simulink model "UART"  (R2025a)
settings: Solver=FixedStepAuto  StartTime=0.0  StopTime=10  FixedStep=1e-6  RelTol=1e-3
undefined symbols (not defined in the file): Bit_1, Bit_2, Bit_3, Bit_4, Bit_5, Bit_6, Bit_7, Bit_8
libraries: simulink_extras x158, fl_lib x17, nesl_utility x8, simulink x7
(part 1 of 6)
settings Model: PacingRate=0.010000  Creator=Erys  LastModifiedBy=Erys
settings SolverCC: AllowMultiTaskInputOutput=on

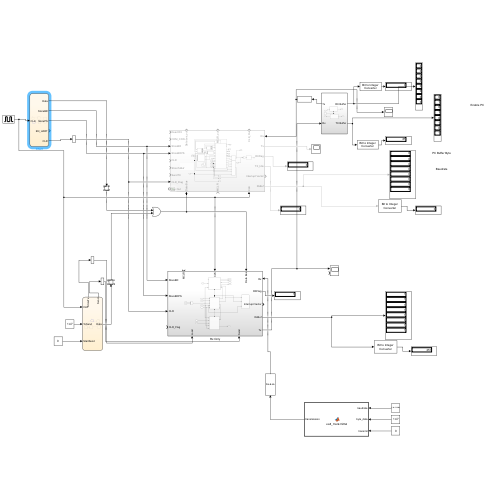
[thumbnail: Simulink's stored preview of the top-level diagram]
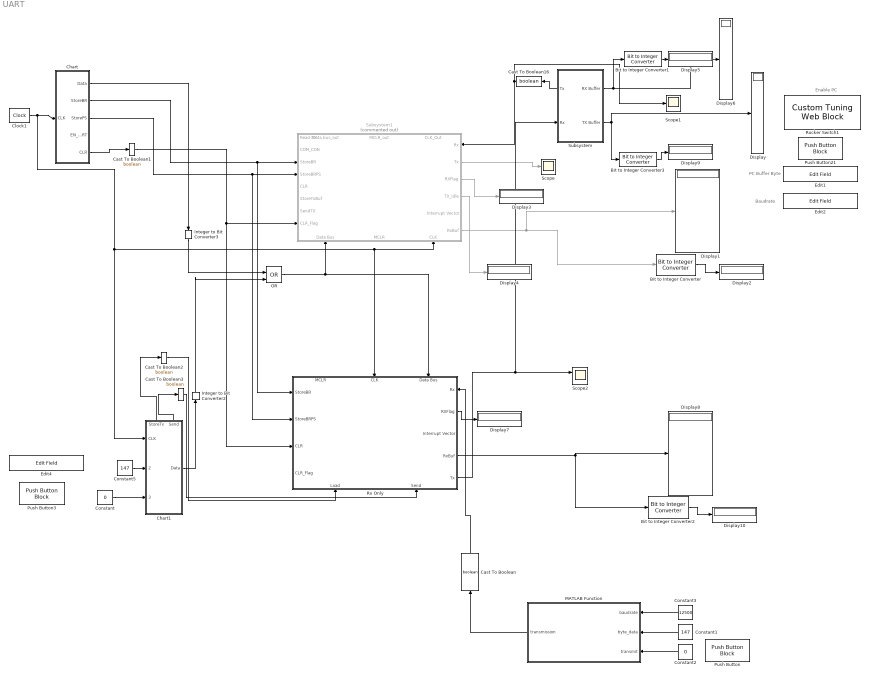
== system UART ==
  note: Enable PC
  note: Baudrate
  note: PC Buffer Byte
  Bit to Integer Converter{,1..3} (4 alike) : simulink/Logic and Bit Operations/Bit to Integer Converter  nbits=8  bitOrder=MSB first  signedOutputValues=Unsigned  outDtype=Inherit via internal rule  outDtypeSigned=Inherit via internal rule
  Cast To Boolean{,1..3,16} (5 alike) : DataTypeConversion  OutDataTypeStr=boolean  SaturateOnIntegerOverflow=off  RndMeth=Floor
  Chart : Stateflow chart  TreatAsAtomicUnit=on
      settings: PortSchema="{\"entries\":[{\"content\":{\"sides\":[{\"content\":{\"connectorIds\":[\"In1\"]},\"type\":\"ConnectorPlacement.EquallySpacedRectSide\",\"uuid\":\"579546ec-ba1d-42e0-bb7d-99479c6f4574\"},{\"content\":{\"connectorIds\":[\"Out2\",\"Out3\",\"Out4\",\"Out5\",\"Out1\"],\"side\":\"RIGHT\"},\"type\":\"ConnectorPlacement.EquallySpacedRectSide\",\"uuid\":\"86ca8068-8b90-4ed4-9903-80afb514b4dd\"},{\"content\":{\"side\":\"TOP\"},\"type\":\"ConnectorPlacement.EquallySpacedRectSide\",\"uuid\":\"acfe83ec-086c-472c-903c-42e246259d52\"}]},\"type\":\"ConnectorPlacement.EquallySpacedConnector\",\"uuid\":\"539fa3bb-c07f-4066-9107-75efb32f7eda\"}],\"packageUris\":[\"http://schema.mathworks.com/mf0/Connector/R2020b\"],\"version\":\"1.0\"}"
  Chart1 : Stateflow chart  TreatAsAtomicUnit=on
      settings: PortSchema="{\"entries\":[{\"content\":{\"sides\":[{\"content\":{\"connectorIds\":[\"In1\",\"In2\",\"In3\"]},\"type\":\"ConnectorPlacement.EquallySpacedRectSide\",\"uuid\":\"579546ec-ba1d-42e0-bb7d-99479c6f4574\"},{\"content\":{\"connectorIds\":[\"Out1\"],\"side\":\"RIGHT\"},\"type\":\"ConnectorPlacement.EquallySpacedRectSide\",\"uuid\":\"86ca8068-8b90-4ed4-9903-80afb514b4dd\"},{\"content\":{\"connectorIds\":[\"Out2\",\"Out3\"],\"side\":\"TOP\"},\"type\":\"ConnectorPlacement.EquallySpacedRectSide\",\"uuid\":\"acfe83ec-086c-472c-903c-42e246259d52\"}]},\"type\":\"ConnectorPlacement.EquallySpacedConnector\",\"uuid\":\"539fa3bb-c07f-4066-9107-75efb32f7eda\"}],\"packageUris\":[\"http://schema.mathworks.com/mf0/Connector/R2020b\"],\"version\":\"1.0\"}"
  Clock1 : simulink_extras/Flip Flops/Clock  period=0.00001
  Constant : Constant  Value=0
  Constant1 : Constant  Value=147
  Constant2 : Constant  Value=0
  Constant3 : Constant  Value=12500
  Constant5 : Constant  Value=147  OutDataTypeStr=double
  Display{,1..10} (11 alike) : Display
  Edit1 : EditField  LabelPosition=Hide  ShowInitialText=on  Alignment=Center
  Edit2 : EditField  LabelPosition=Hide  ShowInitialText=on  Alignment=Center
  Edit4 : EditField  LabelPosition=Hide  ShowInitialText=on  Alignment=Center
  Integer to Bit Converter2 : simulink/Logic and Bit Operations/Integer to Bit Converter  nbits=8  signedInputValues=Unsigned  bitOrder=MSB first  outDtype=Inherit via internal rule
  Integer to Bit Converter3 : simulink/Logic and Bit Operations/Integer to Bit Converter  nbits=8  signedInputValues=Unsigned  bitOrder=MSB first  outDtype=Inherit via internal rule
  MATLAB Function : MATLAB Function  TreatAsAtomicUnit=on
  OR : Logic  Operator=OR  IconShape=distinctive  AllPortsSameDT=off  OutDataTypeStr=boolean
  Push Button : PushButtonBlock  IconOnColor=[0.0, 0.39215686274509803, 0.0]  IconOffColor=[0.0, 1.0, 0.0]  OffValue=0.000000
  Push Button21 : PushButtonBlock  ButtonText=Send  IconOnColor=[0.0, 0.39215686274509803, 0.0]  IconOffColor=[0.0, 1.0, 0.0]  OffValue=0.000000
  Push Button3 : PushButtonBlock  ButtonText=Send  ButtonType=Latch  IconOnColor=[0.0, 0.39215686274509803, 0.0]  IconOffColor=[0.0, 1.0, 0.0]  OffValue=0.000000
  Rocker Switch1 : CustomTuningWebBlock  LabelPosition=Hide  ShowInitialText=on  Configuration="{\"components\":[{\"name\":\"CustomSwitchStateComponent\",\"settings\":{\"position\":[0,0,1,1],\"states\":[{\"HitRegion\":{\"position\":[0,0,0.5,1]},\"Image\":{\"position\":[0.13,0,1,0.75],\"size\":[1,0.75],\"src\":\"data:image\\/svg+xml;base64,PHN2ZyB4bWxucz0iaHR0cDovL3d3dy53My5vcmcvMjAwMC9zdmciIHhtbG5zOnhsaW5rPSJodHRwOi8vd3d3LnczLm9yZy8xOTk5L3hsaW5rIiB2aWV3Qm94PSIwIDAgNzUgMjQuOCI+PGRlZnM+PHN0eWxlPi5jbHMtMXtmaWxsOnVybCgjcmFkaWFsLWdyYWRpZW50KTt9LmNscy0ye2ZpbGw6dXJsKCNyYWRpYWwtZ3JhZGllbnQtMik7fS5jbHMtM3tzdHJva2U6I2IyMDAwMDtzdHJva2Utd2lkdGg6MC4yNXB4O2ZpbGw6dXJsKCNsaW5lYXItZ3JhZGllbnQpO30uY2xzLTR7ZmlsbDp1cmwoI2xpbmVhci1ncmFkaWVudC0yKTt9LmNs ...(+3576 chars)\",\"srcOrientation\":\"Right\"},\"Label\":{\"color\":[0.5019607843137255,0.5019607843137255,0.5019607843137255],\"icon\":{\"size\":[0,0],\"src\":[],\"srcOrientation\":\"Right\"},\"iconPlacement\":\"left\",\"opacity\":1,\"position\":[0.5,0.08],\"show\":true,\"text\":{\"content\":\"Off\",\"font\":\"Helvetica\"}},\"Value\":0},{\"HitRegion\":{\"position\":[0,0.5,0.5,1]},\"Image\":{\"position\":[0.13,0,1,0.75],\"size\":[1,0.75],\"src\":\"data:image\\/svg+xml;base64,PHN2ZyB4bWxucz0iaHR0cDovL3d3dy53My5vcmcvMjAwMC9zdmciIHhtbG5zOnhsaW5rPSJodHRwOi8vd3d3LnczLm9yZy8xOTk5L3hsaW5rIiB2aWV3Qm94PSIwIDAgNzUgMjQuOCI+PGRlZnM+PHN0eWxlPi5jbHMtMXtmaWxsOnVybCgjcmFkaWFsLWdyYWRpZW50KTt9LmNscy0ye2ZpbGw6dXJsKCNyYWRpYWwtZ3JhZGllbnQtMik7fS5jbHMtM3tzdHJva2U6I2IyMDAwMDtzdHJva2Utd2lkdGg6MC4yNXB4O2ZpbGw6dXJsKCNsaW5lYXItZ3JhZGllbnQpO30uY2xzLTR7ZmlsbDp1cmwoI2xpbmVhci1ncmFkaWVudC0yKTt9LmNs ...(+3520 chars)\",\"srcOrientation\":\"Right\"},\"Label\":{\"color\":[0.5019607843137255,0.5019607843137255,0.5019607843137255],\"icon\":{\"size\":[0,0],\"src\":[],\"srcOrientation\":\"Right\"},\"iconPlacement\":\"left\",\"opacity\":1,\"position\":[0.5,0.92],\"show\":true,\"text\":{\"content\":\"On\",\"font\":\"Helvetica\"}},\"Value\":1}]}},{\"name\":\"BackgroundImageComponent\",\"settings\":{\"image\":{\"size\":[155,70],\"src\":\"default\",\"srcOrientation\":\"Right\"},\"position\":[0,0,1,1],\"scaleMode\":\"0\"}},{\"name\":\"ForegroundImageComponent\",\"settings\":{\"image\":{\"size\":[0,0],\"src\":\"default\",\"srcOrientation\":[]},\"isForeground\":1,\"position\":[0,0,1,1],\"scaleMode\":\"0\"}}],\"derived\":{\"blockParameters\":{\"StatesJSON\":[{\"Label\":\"Off\",\"Value\":0},{\"Label\":\"On\",\"Value\":1}],\"fixedAspectRatio\":\"on\"}},\"settings\":{\"BindingType\":\"param\",\"backgroundColor\":[0,0,255,\"1\"],\"backgroundOffset\":0.14,\"fixedAspectRatio\":\"on\",\"foregroundColor\":[234,234,234],\"showBackgroundColor\":false,\"variant\":\"rocker\",\"version\":\"R2024b\"},\"type\":\"Switch\"}"
  Rx Only : Subsystem
      settings: PortSchema="{\"entries\":[{\"content\":{\"sides\":[{\"content\":{\"connectorIds\":[\"In1\",\"In2\",\"In3\",\"In4\"]},\"type\":\"ConnectorPlacement.EquallySpacedRectSide\",\"uuid\":\"e85603b6-4ed5-4461-b09c-fd6c21df1c06\"},{\"content\":{\"connectorIds\":[\"In10\",\"Out1\",\"Out2\",\"Out3\",\"Out4\"],\"side\":\"RIGHT\"},\"type\":\"ConnectorPlacement.EquallySpacedRectSide\",\"uuid\":\"5db2c6ff-63a0-4798-8f8b-4dedc9cdcacf\"},{\"content\":{\"connectorIds\":[\"In5\",\"In6\",\"In7\"],\"side\":\"TOP\"},\"type\":\"ConnectorPlacement.EquallySpacedRectSide\",\"uuid\":\"f0c8188e-88ef-4c96-9e6b-84318d61a16d\"},{\"content\":{\"connectorIds\":[\"In8\",\"In9\"],\"side\":\"BOTTOM\"},\"type\":\"ConnectorPlacement.EquallySpacedRectSide\",\"uuid\":\"72c99dac-0a0c-46d1-ab81-9f63741ecdc0\"}]},\"type\":\"ConnectorPlacement.EquallySpacedConnector\",\"uuid\":\"b744ad23-58d2-4187-a0b7-9a75f0b078d3\"}],\"packageUris\":[\"http://schema.mathworks.com/mf0/Connector/R2020b\"],\"version\":\"1.0\"}"
  Scope : Scope
      settings: ActiveDisplayYMinimum=-1  ActiveDisplayYMaximum=1
  Scope1 : Scope
      settings: ActiveDisplayYMinimum=-0.125  ActiveDisplayYMaximum=1.125
  Scope2 : Scope  NumInputPorts=2
      settings: ActiveDisplayYMinimum=0.9  ActiveDisplayYMaximum=1.1
  Subsystem : Subsystem
      settings: PortSchema="{\"entries\":[{\"content\":{\"sides\":[{\"content\":{\"connectorIds\":[\"Out3\",\"In1\"]},\"type\":\"ConnectorPlacement.EquallySpacedRectSide\",\"uuid\":\"895b9a17-19e6-4759-8585-1efebccf03ce\"},{\"content\":{\"connectorIds\":[\"Out1\",\"Out2\"],\"side\":\"RIGHT\"},\"type\":\"ConnectorPlacement.EquallySpacedRectSide\",\"uuid\":\"c1f476a2-53d3-43a2-8378-f6bf9a8ea71f\"},{\"content\":{\"side\":\"TOP\"},\"type\":\"ConnectorPlacement.EquallySpacedRectSide\",\"uuid\":\"a179f0e6-f4b5-47af-a583-92dca50b06ef\"}]},\"type\":\"ConnectorPlacement.EquallySpacedConnector\",\"uuid\":\"ea5a564d-b62d-4fb1-ae9a-ba3c651dd29f\"}],\"packageUris\":[\"http://schema.mathworks.com/mf0/Connector/R2020b\"],\"version\":\"1.0\"}"
  Subsystem1 : Subsystem  Commented=on
      settings: PortSchema="{\"entries\":[{\"content\":{\"sides\":[{\"content\":{\"connectorIds\":[\"In1\",\"In2\",\"In3\",\"In4\",\"In5\",\"In6\",\"In7\",\"In8\",\"LConn1\"]},\"type\":\"ConnectorPlacement.EquallySpacedRectSide\",\"uuid\":\"e85603b6-4ed5-4461-b09c-fd6c21df1c06\"},{\"content\":{\"connectorIds\":[\"In12\",\"Out1\",\"Out2\",\"Out3\",\"Out4\",\"Out5\"],\"side\":\"RIGHT\"},\"type\":\"ConnectorPlacement.EquallySpacedRectSide\",\"uuid\":\"5db2c6ff-63a0-4798-8f8b-4dedc9cdcacf\"},{\"content\":{\"connectorIds\":[\"Out6\",\"Out7\",\"Out8\"],\"side\":\"TOP\"},\"type\":\"ConnectorPlacement.EquallySpacedRectSide\",\"uuid\":\"f0c8188e-88ef-4c96-9e6b-84318d61a16d\"},{\"content\":{\"connectorIds\":[\"In9\",\"In10\",\"In11\"],\"side\":\"BOTTOM\"},\"type\":\"ConnectorPlacement.EquallySpacedRectSide\",\"uuid\":\"72c99dac-0a0c-46d1-ab81-9f63741ecdc0\"}]},\"type\":\"ConnectorPlacement.EquallySpacedConnector\",\"uuid\":\"b744ad23-58d2-4187-a0b7-9a75f0b078d3\"}],\"packageUris\":[\"http://schema.mathworks.com/mf0/Connector/R2020b\"],\"version\":\"1.0\"}"
  wires:
  Bit to Integer Converter1/1 -> Display5/1
  Subsystem/1(RX Buffer) -> Display6/1, Bit to Integer Converter1/1
  Subsystem/3(Tx) -> Cast To Boolean16/1
  Subsystem/2(TX Buffer) -> Display/1, Bit to Integer Converter3/1
  Bit to Integer Converter3/1 -> Display9/1
  Clock1/1 -> Subsystem1/11(CLK), Rx Only/6(CLK), Chart1/1(CLK), Chart/1(CLK)
  Bit to Integer Converter/1 -> Display2/1
  Subsystem1/5(RxBuf) -> Display1/1, Bit to Integer Converter/1
  Cast To Boolean16/1 -> Subsystem1/12(Rx), Scope1/1
  Chart/3(StoreBR) -> Rx Only/1(StoreBR), Subsystem1/3(StoreBR)
  Chart/4(StorePS) -> Rx Only/2(StoreBRPS), Subsystem1/4(StoreBRPS)
  Chart/1(CLR) -> Cast To Boolean1/1
  Chart1/3(Send) -> Cast To Boolean3/1
  Cast To Boolean1/1 -> Rx Only/3(CLR), Subsystem1/8(CLR_Flag)
  Subsystem1/1(Tx) -> Scope/1
  Chart1/1(Data) -> Integer to Bit Converter2/1
  Chart1/2(StoreTx) -> Cast To Boolean2/1
  Constant5/1 -> Chart1/2(ToSend)
  Constant/1 -> Chart1/3(StartSend)
  Integer to Bit Converter2/1 -> OR/2
  Chart/2(Data) -> Integer to Bit Converter3/1
  OR/1 -> Rx Only/7(Data Bus), Subsystem1/9(Data Bus)
  Integer to Bit Converter3/1 -> OR/1
  Subsystem1/2(RXFlag) -> Display3/1
  Subsystem1/3(TX_Idle) -> Display4/1
  Rx Only/1(RXFlag) -> Display7/1
  Bit to Integer Converter2/1 -> Display10/1
  Rx Only/3(RxBuf) -> Display8/1, Bit to Integer Converter2/1
  Constant1/1 -> MATLAB Function/2(byte_data)
  Constant3/1 -> MATLAB Function/1(baudrate)
  Constant2/1 -> MATLAB Function/3(transmit)
  MATLAB Function/1(transmission) -> Cast To Boolean/1
  Cast To Boolean3/1 -> Rx Only/9(Send)
  Cast To Boolean2/1 -> Rx Only/8(Load)
  Rx Only/4(Tx) -> Scope2/1, Subsystem/1(Rx)
  Cast To Boolean/1 -> Rx Only/10(Rx)

== system UART/Rx Only ==
  StoreBR : Inport
  StoreBRPS : Inport  Port=2
  CLR : Inport  Port=3
  CLR_Flag : Inport  Port=4
  MCLR : Inport  Port=5
  CLK : Inport  Port=6
  Data Bus : Inport  Port=7
  Load : Inport  Port=8
  Send : Inport  Port=9
  Rx : Inport  Port=10
  Baudrate Generator : Subsystem
      settings: PortSchema="{\"entries\":[{\"content\":{\"sides\":[{\"content\":{\"connectorIds\":[\"In1\",\"In2\",\"In3\",\"In4\",\"In5\"]},\"type\":\"ConnectorPlacement.EquallySpacedRectSide\",\"uuid\":\"d194f446-ff7e-400e-97b6-75d09d731b88\"},{\"content\":{\"connectorIds\":[\"Out1\",\"Out2\",\"Out3\",\"Out4\"],\"side\":\"RIGHT\"},\"type\":\"ConnectorPlacement.EquallySpacedRectSide\",\"uuid\":\"c109133b-911d-4f42-82c9-f4bf3d965687\"},{\"content\":{\"connectorIds\":[\"In6\"],\"side\":\"TOP\"},\"type\":\"ConnectorPlacement.EquallySpacedRectSide\",\"uuid\":\"a9d3f627-7d58-48c5-bb3c-ddb572323ed2\"},{\"content\":{\"connectorIds\":[\"In7\"],\"side\":\"BOTTOM\"},\"type\":\"ConnectorPlacement.EquallySpacedRectSide\",\"uuid\":\"95ca91ff-0310-4968-b6f0-040fa48d6210\"}]},\"type\":\"ConnectorPlacement.EquallySpacedConnector\",\"uuid\":\"72d75e6a-49d5-4268-b431-51d3f4095294\"}],\"packageUris\":[\"http://schema.mathworks.com/mf0/Connector/R2020b\"],\"version\":\"1.0\"}"
  OR4 : Logic  Operator=OR  IconShape=distinctive  AllPortsSameDT=off  OutDataTypeStr=boolean
  Scope : Scope  NumInputPorts=3
      settings: ActiveDisplayString=3  ActiveDisplayYMinimum=-0.12499999999999997  ActiveDisplayYMaximum=1.125  DataLoggingVariableName=ScopeData3
  Subsystem1 : Subsystem
      settings: PortSchema="{\"entries\":[{\"content\":{\"sides\":[{\"content\":{\"connectorIds\":[\"In1\",\"In2\",\"In3\"]},\"type\":\"ConnectorPlacement.EquallySpacedRectSide\",\"uuid\":\"26de21f2-c2ce-4306-8005-25e34fc94ef8\"},{\"content\":{\"connectorIds\":[\"Out1\",\"Out2\",\"In4\",\"Out3\",\"In5\",\"In6\"],\"side\":\"RIGHT\"},\"type\":\"ConnectorPlacement.EquallySpacedRectSide\",\"uuid\":\"87f33876-7706-47c8-9618-d671270088cd\"},{\"content\":{\"side\":\"TOP\"},\"type\":\"ConnectorPlacement.EquallySpacedRectSide\",\"uuid\":\"145d03ab-c1b9-4d18-a52c-c9347f9686a8\"},{\"content\":{\"connectorIds\":[\"Out4\"],\"side\":\"BOTTOM\"},\"type\":\"ConnectorPlacement.EquallySpacedRectSide\",\"uuid\":\"eb75dd28-797f-4c73-8962-4db24c637120\"}]},\"type\":\"ConnectorPlacement.EquallySpacedConnector\",\"uuid\":\"6afd2c35-7a81-4ee8-ac82-dba626904bf2\"}],\"packageUris\":[\"http://schema.mathworks.com/mf0/Connector/R2020b\"],\"version\":\"1.0\"}"
  Subsystem2 : Subsystem
      settings: PortSchema="{\"entries\":[{\"content\":{\"sides\":[{\"content\":{\"connectorIds\":[\"In1\",\"In2\",\"In3\",\"In4\",\"In5\"]},\"type\":\"ConnectorPlacement.EquallySpacedRectSide\",\"uuid\":\"1da95ee2-7c6b-483d-95ed-13ac8495d1ed\"},{\"content\":{\"connectorIds\":[\"In6\",\"Out1\"],\"side\":\"RIGHT\"},\"type\":\"ConnectorPlacement.EquallySpacedRectSide\",\"uuid\":\"39299cfc-3cbd-4586-b435-63be24abc51d\"},{\"content\":{\"connectorIds\":[\"Out2\"],\"side\":\"TOP\"},\"type\":\"ConnectorPlacement.EquallySpacedRectSide\",\"uuid\":\"75fe8f74-28fb-448a-b371-b155707b28cf\"}]},\"type\":\"ConnectorPlacement.EquallySpacedConnector\",\"uuid\":\"bfefa0d3-97e8-496e-8e8b-94574003bbd4\"}],\"packageUris\":[\"http://schema.mathworks.com/mf0/Connector/R2020b\"],\"version\":\"1.0\"}"
  RXFlag : Outport
  Interrupt Vector : Outport  Port=2
  RxBuf : Outport  Port=3
  Tx : Outport  Port=4
  wires:
  MCLR/1 -> OR4/2
  OR4/1 -> Subsystem2/1(UARTCLR), Baudrate Generator/3(CLR), Subsystem1/3(UART_CLR)
  CLK/1 -> Scope/3, Baudrate Generator/4(CLK), Subsystem2/4(CLK)
  StoreBRPS/1 -> Baudrate Generator/2(StoreTPS)
  StoreBR/1 -> Baudrate Generator/1(StoreBR)
  Baudrate Generator/2(B_CLK_RX) -> Subsystem1/5(B_CLK), Scope/1  "BAUD CLK"
  CLR/1 -> OR4/1
  Data Bus/1 -> Baudrate Generator/5(Data Bus), Subsystem2/5(Data Bus)
  Send/1 -> Subsystem2/2(SendTX)
  Load/1 -> Subsystem2/3(Load)
  Subsystem2/1(Tx) -> Tx/1
  Baudrate Generator/3(!B_CLK_Tx) -> Subsystem2/6(!B_CLK)
  Rx/1 -> Subsystem1/4(Rx)
  Baudrate Generator/1(!B_CLK_RX) -> Subsystem1/6(!B_CLK)
  CLR_Flag/1 -> Subsystem1/2(CLR_Flag)
  Subsystem1/1(Interrupt Vector) -> Interrupt Vector/1
  Subsystem1/2(Flag) -> RXFlag/1
  Subsystem1/3(RxBuf) -> RxBuf/1
  Subsystem2/2(En_BR) -> Baudrate Generator/7(EnableTx)
  Subsystem1/4(EN_BR) -> Scope/2, Baudrate Generator/6(EnableRx)

== system UART/Subsystem ==
  Rx : Inport
  Constant23 : Constant  Value=12500
  PC RX : Subsystem
      settings: PortSchema="{\"entries\":[{\"content\":{\"sides\":[{\"content\":{\"connectorIds\":[\"In1\"]},\"type\":\"ConnectorPlacement.EquallySpacedRectSide\",\"uuid\":\"5c36fdb9-58e4-4bac-90ea-ae3fb9547746\"},{\"content\":{\"connectorIds\":[\"Out1\"],\"side\":\"RIGHT\"},\"type\":\"ConnectorPlacement.EquallySpacedRectSide\",\"uuid\":\"305a7217-1c2b-4e42-91b3-038d16c5c055\"},{\"content\":{\"side\":\"TOP\"},\"type\":\"ConnectorPlacement.EquallySpacedRectSide\",\"uuid\":\"8bca033e-7423-4813-979e-646ac4ffc9f5\"},{\"content\":{\"connectorIds\":[\"In2\"],\"side\":\"BOTTOM\"},\"type\":\"ConnectorPlacement.EquallySpacedRectSide\",\"uuid\":\"0fb3eda9-6a9e-42f2-8b90-ae90f87eee38\"}]},\"type\":\"ConnectorPlacement.EquallySpacedConnector\",\"uuid\":\"4522f435-3b11-47d6-b8b1-c58661572e67\"}],\"packageUris\":[\"http://schema.mathworks.com/mf0/Connector/R2020b\"],\"version\":\"1.0\"}"
  PC Tx : Subsystem
      settings: PortSchema="{\"entries\":[{\"content\":{\"sides\":[{\"content\":{\"connectorIds\":[\"Out2\"]},\"type\":\"ConnectorPlacement.EquallySpacedRectSide\",\"uuid\":\"4cc81552-4785-4fe1-ba4c-afd427c4a9be\"},{\"content\":{\"connectorIds\":[\"Out1\"],\"side\":\"RIGHT\"},\"type\":\"ConnectorPlacement.EquallySpacedRectSide\",\"uuid\":\"17a0d90d-16da-439e-9c28-79f860db0d72\"},{\"content\":{\"connectorIds\":[\"In1\"],\"side\":\"TOP\"},\"type\":\"ConnectorPlacement.EquallySpacedRectSide\",\"uuid\":\"85a74a21-901d-48e2-982c-d40d9a6c8828\"}]},\"type\":\"ConnectorPlacement.EquallySpacedConnector\",\"uuid\":\"f7431681-2562-4b57-bc58-81cf5712b5b5\"}],\"packageUris\":[\"http://schema.mathworks.com/mf0/Connector/R2020b\"],\"version\":\"1.0\"}"
  RX Buffer : Outport
  TX Buffer : Outport  Port=2
  Tx : Outport  Port=3
  wires:
  Rx/1 -> PC RX/1(Rx)
  PC Tx/2(Tx) -> Tx/1
  PC RX/1(Buffer) -> RX Buffer/1
  PC Tx/1(Buffer) -> TX Buffer/1
  Constant23/1 -> PC Tx/1(Baudrate), PC RX/2(Baudrate)

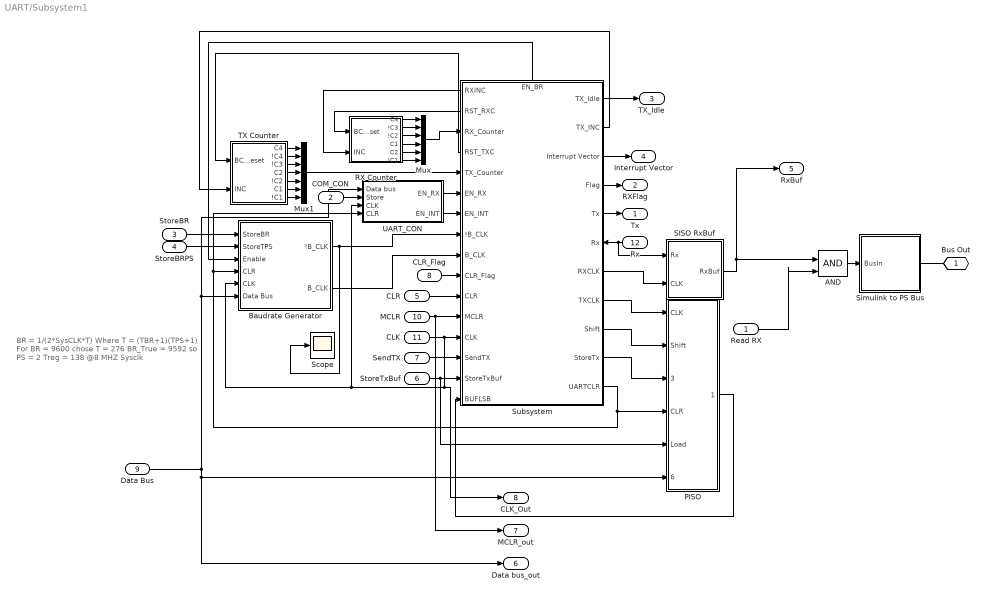
== system UART/Subsystem1 ==
  note: BR = 1/(2*SysCLK*T)
      | Where T = (TBR+1)(TPS+1)
      | For BR = 9600 chose T = 276 BR_True = 9592
      |
      | so PS = 2
      | Treg = 138
      |
      | @8 MHZ Sysclk
  Read RX : Inport
  COM_CON : Inport  Port=2
  StoreBR : Inport  Port=3
  StoreBRPS : Inport  Port=4
  CLR : Inport  Port=5
  StoreTxBuf : Inport  Port=6
  SendTX : Inport  Port=7
  CLR_Flag : Inport  Port=8
  Data Bus : Inport  Port=9
  MCLR : Inport  Port=10
  CLK : Inport  Port=11
  Rx : Inport  Port=12
  AND : Logic  IconShape=distinctive  AllPortsSameDT=off  OutDataTypeStr=boolean
  Baudrate Generator : Subsystem
  Mux : Mux  Inputs=6
  Mux1 : Mux  Inputs=7
  PISO : Subsystem
  RX Counter : Subsystem
  SISO RxBuf : Subsystem
  Scope : Scope
      settings: ActiveDisplayYMinimum=-0.011295344536901064  ActiveDisplayYMaximum=1.0251315467449829
  Simulink to PS Bus : Subsystem
  Subsystem : Subsystem
      settings: PortSchema="{\"entries\":[{\"content\":{\"sides\":[{\"content\":{\"connectorIds\":[\"Out12\",\"Out13\",\"In1\",\"Out14\",\"In2\",\"In3\",\"In4\",\"In5\",\"In6\",\"In7\",\"In8\",\"In9\",\"In10\",\"In11\",\"In12\",\"In13\"]},\"type\":\"ConnectorPlacement.EquallySpacedRectSide\",\"uuid\":\"5f740d6e-15c2-47b5-8101-a8ac2908b9d5\"},{\"content\":{\"connectorIds\":[\"Out1\",\"Out2\",\"Out3\",\"Out4\",\"Out5\",\"In14\",\"Out6\",\"Out7\",\"Out8\",\"Out9\",\"Out10\"],\"side\":\"RIGHT\"},\"type\":\"ConnectorPlacement.EquallySpacedRectSide\",\"uuid\":\"5d214534-1223-4301-a5a7-3ca5e7f086fd\"},{\"content\":{\"connectorIds\":[\"Out11\"],\"side\":\"TOP\"},\"type\":\"ConnectorPlacement.EquallySpacedRectSide\",\"uuid\":\"1d2213ce-2390-4a69-a57b-c28668a5aa5c\"}]},\"type\":\"ConnectorPlacement.EquallySpacedConnector\",\"uuid\":\"5a906a9e-6d2c-4523-95ab-0413fe814690\"}],\"packageUris\":[\"http://schema.mathworks.com/mf0/Connector/R2020b\"],\"version\":\"1.0\"}"
  TX Counter : Subsystem
  UART_CON : Subsystem
  Bus Out : PMIOPort  Side=Left
  Tx : Outport
  RXFlag : Outport  Port=2
  TX_Idle : Outport  Port=3
  Interrupt Vector : Outport  Port=4
  RxBuf : Outport  Port=5
  Data bus_out : Outport  Port=6
  MCLR_out : Outport  Port=7
  CLK_Out : Outport  Port=8
  wires:
  MCLR/1 -> MCLR_out/1, Subsystem/9(MCLR)
  UART_CON/1(EN_RX) -> Subsystem/3(EN_RX)
  UART_CON/2(EN_INT) -> Subsystem/4(EN_INT)
  COM_CON/1 -> UART_CON/2(Store)
  SendTX/1 -> Subsystem/11(SendTX)
  CLR_Flag/1 -> Subsystem/7(CLR_Flag)
  Data Bus/1 -> PISO/6(Data Bus), Data bus_out/1, Baudrate Generator/6(Data Bus), UART_CON/1(Data bus)
  StoreTxBuf/1 -> Subsystem/12(StoreTxBuf), PISO/5(Load)
  Subsystem/13(RST_RXC) -> RX Counter/1(BC_Reset)
  Subsystem/9(StoreTx) -> PISO/3(Store TXBUF)
  Subsystem/2(TX_INC) -> TX Counter/2(INC)
  Subsystem/14(RST_TXC) -> TX Counter/1(BC_Reset)
  Subsystem/4(Flag) -> RXFlag/1
  Subsystem/3(Interrupt Vector) -> Interrupt Vector/1
  Subsystem/12(RXINC) -> RX Counter/2(INC)
  Subsystem/10(UARTCLR) -> UART_CON/4(CLR), Baudrate Generator/4(CLR), PISO/4("CLR ")
  Rx/1 -> SISO RxBuf/1(Rx), Subsystem/14(Rx)
  CLK/1 -> Subsystem/10(CLK), CLK_Out/1, Baudrate Generator/5(CLK), UART_CON/3(CLK)
  Subsystem/5(Tx) -> Tx/1
  Subsystem/7(TXCLK) -> PISO/1("CLK ")
  Subsystem/11(EN_BR) -> Baudrate Generator/3(Enable)
  Subsystem/8(Shift) -> PISO/2(Shift)
  StoreBRPS/1 -> Baudrate Generator/2(StoreTPS)
  StoreBR/1 -> Baudrate Generator/1(StoreBR)
  SISO RxBuf/1(RxBuf) -> RxBuf/1, AND/1
  PISO/1(Serial_out) -> Subsystem/13(BUFLSB)
  Baudrate Generator/2(B_CLK) -> Subsystem/6(B_CLK)
  Baudrate Generator/1(!B_CLK) -> Scope/1, Subsystem/5(!B_CLK)
  RX Counter/1(C4) -> Mux/1
  RX Counter/2(!C3) -> Mux/2
  RX Counter/3(!C2) -> Mux/3
  RX Counter/4(C1) -> Mux/4
  Mux/1 -> Subsystem/1(RX_Counter)
  TX Counter/1(C4) -> Mux1/1
  TX Counter/2(!C4) -> Mux1/2
  TX Counter/3(!C3) -> Mux1/3
  TX Counter/4(C2) -> Mux1/4
  TX Counter/5(!C2) -> Mux1/5
  TX Counter/6(C1) -> Mux1/6
  TX Counter/7(!C1) -> Mux1/7
  Mux1/1 -> Subsystem/2(TX_Counter)
  CLR/1 -> Subsystem/8(CLR)
  Subsystem/1(TX_Idle) -> TX_Idle/1
  Read RX/1 -> AND/2
  AND/1 -> Simulink to PS Bus/1(BusIn)
  RX Counter/5(C2) -> Mux/5
  RX Counter/6(!C1) -> Mux/6
  Subsystem/6(RXCLK) -> SISO RxBuf/2(CLK)
  connections:
  Bus Out/RConn1 -- Simulink to PS Bus/RConn1

== system UART/Rx Only/Baudrate Generator ==
  StoreBR : Inport
  StoreTPS : Inport  Port=2
  CLR : Inport  Port=3
  CLK : Inport  Port=4
  Data Bus : Inport  Port=5
  EnableRx : Inport  Port=6
  EnableTx : Inport  Port=7
  BPS : Subsystem
  BR : Subsystem
  BaudTimer : Subsystem
  BaudTimer1 : Subsystem
  !B_CLK_RX : Outport
  B_CLK_RX : Outport  Port=2
  !B_CLK_Tx : Outport  Port=3
  B_CLK_Tx : Outport  Port=4
  wires:
  CLK/1 -> BaudTimer/7(CLK), BaudTimer1/7(CLK), BR/3(CLK), BPS/3(CLK)
  StoreBR/1 -> BaudTimer/1(StoreBR), BaudTimer1/1(StoreBR), BR/2(Store)
  Data Bus/1 -> BPS/1(Data bus), BR/1(Data bus)
  CLR/1 -> BaudTimer1/4("CLR "), BPS/4(CLR), BaudTimer/4("CLR "), BR/4(CLR)
  StoreTPS/1 -> BaudTimer/5(StorePS), BaudTimer1/5(StorePS), BPS/2(Store)
  BR/1("Q Bus ") -> BaudTimer/2(BR_Reg), BaudTimer1/2(BR_Reg)
  EnableRx/1 -> BaudTimer/3(Enable)
  BPS/1("Q Bus ") -> BaudTimer/6(TReg), BaudTimer1/6(TReg)
  BaudTimer/2(!B_CLK) -> !B_CLK_RX/1
  BaudTimer/1(B_CLK) -> B_CLK_RX/1
  EnableTx/1 -> BaudTimer1/3(Enable)
  BaudTimer1/2(!B_CLK) -> !B_CLK_Tx/1
  BaudTimer1/1(B_CLK) -> B_CLK_Tx/1

== system UART/Rx Only/Subsystem1 ==
  EN_INT : Inport
  CLR_Flag : Inport  Port=2
  UART_CLR : Inport  Port=3
  Rx : Inport  Port=4
  B_CLK : Inport  Port=5
  !B_CLK : Inport  Port=6
  Constant : Constant
  Mux : Mux
  RX Counter : Subsystem
  SIPO RxBuf : Subsystem
  Subsystem : Subsystem
      settings: PortSchema="{\"entries\":[{\"content\":{\"sides\":[{\"content\":{\"connectorIds\":[\"Out5\",\"Out6\",\"In1\",\"In2\",\"In3\",\"In4\",\"In5\",\"In6\"]},\"type\":\"ConnectorPlacement.EquallySpacedRectSide\",\"uuid\":\"5f740d6e-15c2-47b5-8101-a8ac2908b9d5\"},{\"content\":{\"connectorIds\":[\"Out1\",\"Out2\",\"In8\",\"Out3\"],\"side\":\"RIGHT\"},\"type\":\"ConnectorPlacement.EquallySpacedRectSide\",\"uuid\":\"5d214534-1223-4301-a5a7-3ca5e7f086fd\"},{\"content\":{\"connectorIds\":[\"Out4\"],\"side\":\"TOP\"},\"type\":\"ConnectorPlacement.EquallySpacedRectSide\",\"uuid\":\"1d2213ce-2390-4a69-a57b-c28668a5aa5c\"},{\"content\":{\"connectorIds\":[\"In7\"],\"side\":\"BOTTOM\"},\"type\":\"ConnectorPlacement.EquallySpacedRectSide\",\"uuid\":\"8027d3ec-90e1-4e8c-832f-866f1decbd3b\"}]},\"type\":\"ConnectorPlacement.EquallySpacedConnector\",\"uuid\":\"5a906a9e-6d2c-4523-95ab-0413fe814690\"}],\"packageUris\":[\"http://schema.mathworks.com/mf0/Connector/R2020b\"],\"version\":\"1.0\"}"
  Interrupt Vector : Outport
  Flag : Outport  Port=2
  RxBuf : Outport  Port=3
  EN_BR : Outport  Port=4
  wires:
  Rx/1 -> SIPO RxBuf/1(Rx), Subsystem/8(Rx)
  Constant/1 -> Subsystem/2(EN_RX)
  Subsystem/5(RXINC) -> RX Counter/2(INC)
  EN_INT/1 -> Subsystem/3(EN_INT)
  Subsystem/2(Flag) -> Flag/1
  RX Counter/2(!C3) -> Mux/2
  RX Counter/3(!C2) -> Mux/3
  RX Counter/4(C1) -> Mux/4
  Subsystem/3(RXCLK) -> SIPO RxBuf/2(CLK)
  Subsystem/4(EN_BR) -> EN_BR/1
  RX Counter/1(C4) -> Mux/1
  Subsystem/6(RST_RXC) -> RX Counter/1(BC_Reset)
  Mux/1 -> Subsystem/1(RX_Counter)
  UART_CLR/1 -> Subsystem/7(UART_CLR)
  !B_CLK/1 -> Subsystem/4(!B_CLK)
  Subsystem/1(Interrupt Vector) -> Interrupt Vector/1
  SIPO RxBuf/1(RxBuf) -> RxBuf/1
  CLR_Flag/1 -> Subsystem/6(CLR_Flag)
  B_CLK/1 -> Subsystem/5(B_CLK)

== system UART/Rx Only/Subsystem2 ==
  UARTCLR : Inport
  SendTX : Inport  Port=2
  Load : Inport  Port=3
  CLK : Inport  Port=4
  Data Bus : Inport  Port=5
  !B_CLK : Inport  Port=6
  Mux1 : Mux
  PISO : Subsystem
      settings: PortSchema="{\"entries\":[{\"content\":{\"sides\":[{\"content\":{\"connectorIds\":[\"In1\",\"In2\",\"Out1\",\"In3\",\"In4\"]},\"type\":\"ConnectorPlacement.EquallySpacedRectSide\",\"uuid\":\"1a70dc94-6fd8-45e6-a964-690408e545a5\"},{\"content\":{\"side\":\"RIGHT\"},\"type\":\"ConnectorPlacement.EquallySpacedRectSide\",\"uuid\":\"0446f59e-5565-4f21-b86e-aa6a6c358594\"},{\"content\":{\"connectorIds\":[\"In5\",\"In6\"],\"side\":\"TOP\"},\"type\":\"ConnectorPlacement.EquallySpacedRectSide\",\"uuid\":\"b3251efb-1b02-4ea6-9880-a7aeacd90048\"}]},\"type\":\"ConnectorPlacement.EquallySpacedConnector\",\"uuid\":\"49ea71c8-7b9a-4520-8019-77c12bbc3963\"}],\"packageUris\":[\"http://schema.mathworks.com/mf0/Connector/R2020b\"],\"version\":\"1.0\"}"
  RX Counter1 : Subsystem
  Subsystem1 : Subsystem
      settings: PortSchema="{\"entries\":[{\"content\":{\"sides\":[{\"content\":{\"connectorIds\":[\"Out5\",\"Out6\",\"In1\",\"In2\",\"In3\",\"In4\",\"In5\"]},\"type\":\"ConnectorPlacement.EquallySpacedRectSide\",\"uuid\":\"5f740d6e-15c2-47b5-8101-a8ac2908b9d5\"},{\"content\":{\"connectorIds\":[\"Out1\",\"Out2\",\"Out3\",\"In7\"],\"side\":\"RIGHT\"},\"type\":\"ConnectorPlacement.EquallySpacedRectSide\",\"uuid\":\"5d214534-1223-4301-a5a7-3ca5e7f086fd\"},{\"content\":{\"connectorIds\":[\"In6\",\"Out4\"],\"side\":\"TOP\"},\"type\":\"ConnectorPlacement.EquallySpacedRectSide\",\"uuid\":\"1d2213ce-2390-4a69-a57b-c28668a5aa5c\"}]},\"type\":\"ConnectorPlacement.EquallySpacedConnector\",\"uuid\":\"5a906a9e-6d2c-4523-95ab-0413fe814690\"}],\"packageUris\":[\"http://schema.mathworks.com/mf0/Connector/R2020b\"],\"version\":\"1.0\"}"
  Tx : Outport
  En_BR : Outport  Port=2
  wires:
  Subsystem1/5(TX_INC) -> RX Counter1/2(INC)
  Load/1 -> PISO/3(Load), Subsystem1/5(Load)
  RX Counter1/3(C2) -> Mux1/3
  RX Counter1/4(C1) -> Mux1/4
  RX Counter1/2(!C3) -> Mux1/2
  Subsystem1/2(TXCLK) -> PISO/1("TXCLK ")
  PISO/1(Serial_out) -> Subsystem1/7(BUFLSB)
  UARTCLR/1 -> Subsystem1/6(UARTCLR), PISO/6("CLR ")
  Subsystem1/4(EN_BR) -> En_BR/1, PISO/5(Shift)
  Subsystem1/3(StoreTx) -> PISO/2(Store TXBUF)
  Mux1/1 -> Subsystem1/1(TX_Counter)
  Subsystem1/6(TXC_RST) -> RX Counter1/1(BC_Reset)
  RX Counter1/1(C4) -> Mux1/1
  SendTX/1 -> Subsystem1/4(SendTX)
  !B_CLK/1 -> Subsystem1/3(!B_CLK)
  Data Bus/1 -> PISO/4(Data Bus)
  Subsystem1/1(Tx) -> Tx/1
  CLK/1 -> Subsystem1/2(CLK)

== system UART/Subsystem/PC RX ==
  Rx : Inport
  Baudrate : Inport  Port=2
  Chart : Stateflow chart  TreatAsAtomicUnit=on
      settings: PortSchema="{\"entries\":[{\"content\":{\"sides\":[{\"content\":{\"connectorIds\":[\"In2\",\"In3\"]},\"type\":\"ConnectorPlacement.EquallySpacedRectSide\",\"uuid\":\"b3a5cf11-253b-48e1-b27d-ab3568105f2d\"},{\"content\":{\"connectorIds\":[\"Out1\"],\"side\":\"RIGHT\"},\"type\":\"ConnectorPlacement.EquallySpacedRectSide\",\"uuid\":\"d77e3c4d-b760-45fc-afb9-9b4c779c0c28\"},{\"content\":{\"side\":\"TOP\"},\"type\":\"ConnectorPlacement.EquallySpacedRectSide\",\"uuid\":\"3ac6c7a6-9511-4efe-9c6f-68eb6d23e231\"},{\"content\":{\"connectorIds\":[\"In1\"],\"side\":\"BOTTOM\"},\"type\":\"ConnectorPlacement.EquallySpacedRectSide\",\"uuid\":\"e6165016-b8f7-4206-b89f-4a6ce8b56855\"}]},\"type\":\"ConnectorPlacement.EquallySpacedConnector\",\"uuid\":\"e620c1e0-2324-4d91-a922-d923d05fb9d1\"}],\"packageUris\":[\"http://schema.mathworks.com/mf0/Connector/R2020b\"],\"version\":\"1.0\"}"
  Constant24 : Constant
  MATLAB Function : MATLAB Function  TreatAsAtomicUnit=on
  Buffer : Outport
  wires:
  MATLAB Function/1(y) -> Chart/1(Baudrate)
  Baudrate/1 -> MATLAB Function/1(u)
  Rx/1 -> Chart/3(Rx)
  Constant24/1 -> Chart/2(Enable)
  Chart/1(Buffer) -> Buffer/1

== system UART/Subsystem/PC Tx ==
  Baudrate : Inport
  Chart : Stateflow chart  TreatAsAtomicUnit=on
      settings: PortSchema="{\"entries\":[{\"content\":{\"sides\":[{\"content\":{\"connectorIds\":[\"In2\",\"In3\",\"In1\"]},\"type\":\"ConnectorPlacement.EquallySpacedRectSide\",\"uuid\":\"0fdeee4d-f616-4de4-9957-3fe333ba6b50\"},{\"content\":{\"connectorIds\":[\"Out1\"],\"side\":\"RIGHT\"},\"type\":\"ConnectorPlacement.EquallySpacedRectSide\",\"uuid\":\"b9b055cb-ef8e-482e-98e8-65c3605d7f8f\"},{\"content\":{\"connectorIds\":[\"In4\"],\"side\":\"TOP\"},\"type\":\"ConnectorPlacement.EquallySpacedRectSide\",\"uuid\":\"a4fa0ffa-46c2-4446-908b-2de4127fdb17\"}]},\"type\":\"ConnectorPlacement.EquallySpacedConnector\",\"uuid\":\"eba70a97-dbbd-4797-9708-a070df84da02\"}],\"packageUris\":[\"http://schema.mathworks.com/mf0/Connector/R2020b\"],\"version\":\"1.0\"}"
  Constant21 : Constant  Value=85
  Constant22 : Constant  Value=0  OutDataTypeStr=boolean
  Constant24 : Constant
  Integer to Bit Converter : simulink/Logic and Bit Operations/Integer to Bit Converter  nbits=8  signedInputValues=Unsigned  bitOrder=MSB first  outDtype=Inherit via internal rule
  MATLAB Function : MATLAB Function  TreatAsAtomicUnit=on
  Buffer : Outport
  Tx : Outport  Port=2
  wires:
  Constant21/1 -> Integer to Bit Converter/1
  Integer to Bit Converter/1 -> Buffer/1, Chart/3(Bits)
  MATLAB Function/1(y) -> Chart/1(Baudrate)
  Constant22/1 -> Chart/2(Send)
  Constant24/1 -> Chart/4(Enable)
  Chart/1(Tx) -> Tx/1
  Baudrate/1 -> MATLAB Function/1(u)

== system UART/Subsystem1/Baudrate Generator ==
  StoreBR : Inport
  StoreTPS : Inport  Port=2
  Enable : Inport  Port=3
  CLR : Inport  Port=4
  CLK : Inport  Port=5
  Data Bus : Inport  Port=6
  BPS : Subsystem
  BR : Subsystem
  Counter : Subsystem
      settings: PortSchema="{\"entries\":[{\"content\":{\"sides\":[{\"content\":{\"connectorIds\":[\"Out1\",\"In1\",\"In2\"]},\"type\":\"ConnectorPlacement.EquallySpacedRectSide\",\"uuid\":\"d2ca064e-8e65-4383-9509-923487f0994b\"},{\"content\":{\"side\":\"RIGHT\"},\"type\":\"ConnectorPlacement.EquallySpacedRectSide\",\"uuid\":\"c8a688a5-ee2c-4fad-a889-c5e09b1c269e\"},{\"content\":{\"side\":\"TOP\"},\"type\":\"ConnectorPlacement.EquallySpacedRectSide\",\"uuid\":\"2f0d42e7-9a85-4a58-8ec6-3b7b9eab62de\"},{\"content\":{\"side\":\"BOTTOM\"},\"type\":\"ConnectorPlacement.EquallySpacedRectSide\",\"uuid\":\"38510fd4-2d07-404d-8bb1-895f71011c48\"}]},\"type\":\"ConnectorPlacement.EquallySpacedConnector\",\"uuid\":\"c9cdc40f-5296-4098-a99e-74109d120565\"}],\"packageUris\":[\"http://schema.mathworks.com/mf0/Connector/R2020b\"],\"version\":\"1.0\"}"
  Counter1 : Subsystem
      settings: PortSchema="{\"entries\":[{\"content\":{\"sides\":[{\"content\":{\"connectorIds\":[\"Out1\",\"In1\",\"In2\"]},\"type\":\"ConnectorPlacement.EquallySpacedRectSide\",\"uuid\":\"d2ca064e-8e65-4383-9509-923487f0994b\"},{\"content\":{\"side\":\"RIGHT\"},\"type\":\"ConnectorPlacement.EquallySpacedRectSide\",\"uuid\":\"c8a688a5-ee2c-4fad-a889-c5e09b1c269e\"},{\"content\":{\"side\":\"TOP\"},\"type\":\"ConnectorPlacement.EquallySpacedRectSide\",\"uuid\":\"2f0d42e7-9a85-4a58-8ec6-3b7b9eab62de\"},{\"content\":{\"side\":\"BOTTOM\"},\"type\":\"ConnectorPlacement.EquallySpacedRectSide\",\"uuid\":\"38510fd4-2d07-404d-8bb1-895f71011c48\"}]},\"type\":\"ConnectorPlacement.EquallySpacedConnector\",\"uuid\":\"c9cdc40f-5296-4098-a99e-74109d120565\"}],\"packageUris\":[\"http://schema.mathworks.com/mf0/Connector/R2020b\"],\"version\":\"1.0\"}"
  Prescaler_Controller1 : Subsystem
      settings: PortSchema="{\"entries\":[{\"content\":{\"sides\":[{\"content\":{\"connectorIds\":[\"In1\",\"In2\",\"In3\",\"In4\",\"In5\"]},\"type\":\"ConnectorPlacement.EquallySpacedRectSide\",\"uuid\":\"82b85bc6-964b-49ee-8a4b-3356bfec1aee\"},{\"content\":{\"connectorIds\":[\"Out1\",\"In6\",\"Out2\",\"Out3\"],\"side\":\"RIGHT\"},\"type\":\"ConnectorPlacement.EquallySpacedRectSide\",\"uuid\":\"8c4af632-7d6e-4ec6-a03e-f6796e56340c\"},{\"content\":{\"side\":\"TOP\"},\"type\":\"ConnectorPlacement.EquallySpacedRectSide\",\"uuid\":\"c668d65a-8355-4e30-8ca9-8213ac4eb35c\"},{\"content\":{\"side\":\"BOTTOM\"},\"type\":\"ConnectorPlacement.EquallySpacedRectSide\",\"uuid\":\"7e82bb91-fecf-4aec-a971-3b22643d51d5\"}]},\"type\":\"ConnectorPlacement.EquallySpacedConnector\",\"uuid\":\"0a0bd963-09d6-4454-bda2-144190581a2a\"}],\"packageUris\":[\"http://schema.mathworks.com/mf0/Connector/R2020b\"],\"version\":\"1.0\"}"
  TController : Subsystem
      settings: PortSchema="{\"entries\":[{\"content\":{\"sides\":[{\"content\":{\"connectorIds\":[\"In1\",\"In2\",\"In3\",\"In4\",\"In5\"]},\"type\":\"ConnectorPlacement.EquallySpacedRectSide\",\"uuid\":\"82b85bc6-964b-49ee-8a4b-3356bfec1aee\"},{\"content\":{\"connectorIds\":[\"In6\",\"Out1\",\"Out2\",\"Out3\",\"Out4\"],\"side\":\"RIGHT\"},\"type\":\"ConnectorPlacement.EquallySpacedRectSide\",\"uuid\":\"8c4af632-7d6e-4ec6-a03e-f6796e56340c\"},{\"content\":{\"side\":\"TOP\"},\"type\":\"ConnectorPlacement.EquallySpacedRectSide\",\"uuid\":\"c668d65a-8355-4e30-8ca9-8213ac4eb35c\"},{\"content\":{\"side\":\"BOTTOM\"},\"type\":\"ConnectorPlacement.EquallySpacedRectSide\",\"uuid\":\"7e82bb91-fecf-4aec-a971-3b22643d51d5\"}]},\"type\":\"ConnectorPlacement.EquallySpacedConnector\",\"uuid\":\"0a0bd963-09d6-4454-bda2-144190581a2a\"}],\"packageUris\":[\"http://schema.mathworks.com/mf0/Connector/R2020b\"],\"version\":\"1.0\"}"
  !B_CLK : Outport
  B_CLK : Outport  Port=2
  wires:
  CLK/1 -> BR/3(CLK), BPS/3(CLK), Prescaler_Controller1/5(CLK)
  Counter/1(TC) -> TController/6(TC)
  TController/1(INC) -> Counter/1(INC)
  TController/3(B_CLK) -> B_CLK/1
  StoreBR/1 -> TController/1(StoreTH), BR/2(Store)
  BR/1("Q Bus ") -> TController/2(TH_Reg)
  Data Bus/1 -> BPS/1(Data bus), BR/1(Data bus)
  CLR/1 -> BR/4(CLR), BPS/4(CLR), Prescaler_Controller1/1("CLR "), TController/3("CLR ")
  Prescaler_Controller1/2(INC) -> Counter1/1(INC)
  Prescaler_Controller1/1(CLK_Next) -> TController/5(CLK)
  Prescaler_Controller1/3(TC_RST) -> Counter1/2(TC_RST)
  StoreTPS/1 -> Prescaler_Controller1/4(StoreTReg), BPS/2(Store)
  BPS/1("Q Bus ") -> Prescaler_Controller1/2(TReg)
  Counter1/1(TC) -> Prescaler_Controller1/6(TC)
  Enable/1 -> Prescaler_Controller1/3(Enable), TController/4(Enable)
  TController/2(TC_RST) -> Counter/2(TC_RST)
  TController/4(!B_CLK) -> !B_CLK/1
